simulink model "adc_nonlinconfig"  (R2013a)
settings: Solver=ode45  StartTime=0.0  StopTime=10e-05  RelTol=1e-3
undefined symbols (not defined in the file or in its folder): One, sided
libraries: dsparch4 x2, nonlinlib_config x1, dspsnks4 x1
settings Model: Creator=bbhattac  LastModifiedBy=bbhattac
settings OptimizationCC: ExpressionDepthLimit=2147483647
settings DebuggingCC: ParameterPrecisionLossMsg=none  FcnCallInpInsideContextMsg=UseLocalSettings
settings GRTTargetCC: CombineOutputUpdateFcns=off  GRTInterface=on

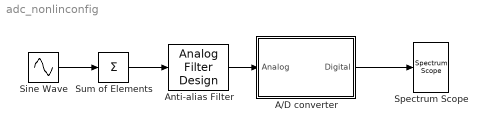
== system adc_nonlinconfig ==
  A/D converter : Subsystem
  Anti-alias Filter : dsparch4/Analog Filter Design  method=Butterworth  filttype=Lowpass  N=8  Wlo=2*pi*50e+06  Whi=80  Rp=2  Rs=40
  Sine Wave : Sin  Amplitude=.5  Frequency=2*pi*[20 22]*1e6  SampleTime=0
  Spectrum Scope : dspsnks4/Spectrum Scope  ScopeProperties=on  Domain=Frequency  HorizSpan=1  UseBuffer=on  BufferSize=2048  Overlap=0  TreatMby1Signals=M channels  inpFftLenInherit=off  FFTlength=128  numAvg=2  DisplayProperties=off  AxisGrid=on  Memory=off  FrameNumber=on  AxisLegend=off  AxisZoom=off  OpenScopeAtSimStart=on  OpenScopeImmediately=off  FigPos=[13 485 399 237]  AxisProperties=off  XUnits=Hertz  XRange=One-sided ([0...Fs/2])  XDisplay=0  InheritXIncr=on  XIncr=1.0  XLabel=Samples  XLimit=Auto  YUnits=dBW/Hertz  XMax=1  XMin=0  YLabel=Magnitude-squared, dB  LineProperties=off  wintypeSpecScope=Hann  RsSpecScope=50  betaSpecScope=5  winsampSpecScope=Periodic  XAxisParamsVer=6.9  isFrameUpgraded=on
      settings: YMin=-146.5665  YMax=-53.7967
  Sum of Elements : Sum  Inputs=+
  wires:
  Sine Wave/1 -> Sum of Elements/1
  Sum of Elements/1 -> Anti-alias Filter/1
  Anti-alias Filter/1 -> A/D converter/1(Analog)
  A/D converter/1(Digital) -> Spectrum Scope/1

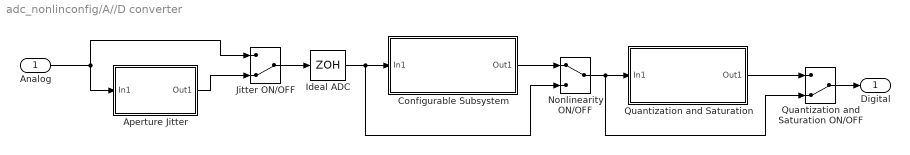
== system adc_nonlinconfig/A//D converter ==
  Analog : Inport
  Aperture Jitter : Subsystem
  Configurable Subsystem : Subsystem  BlockChoice=Lookup Table
      link override Nonlinearity-Sine: nonlingain=0.2
      link override Power Series Nonlinearity: nonlingain=1e-03
      settings: AttributesFormatString=%<BlockChoice>  TemplateBlock=nonlinlib_config/Configurable Subsystem  MemberBlocks=Dead Zone,Lookup Table,Nonlinearity-Sine,Nonlinearity-Tanh,Power Series Nonlinearity
  Ideal ADC : ZeroOrderHold  SampleTime=1/100e6
  Jitter ON/OFF : ManualSwitch  CurrentSetting=0
  Nonlinearity ON/OFF : ManualSwitch
  Quantization and Saturation ON/OFF : ManualSwitch  CurrentSetting=0
  Quantization and Saturation : Subsystem
  Digital : Outport
  wires:
  Analog/1 -> Jitter ON/OFF/1, Aperture Jitter/1(In1)
  Jitter ON/OFF/1 -> Ideal ADC/1
  Ideal ADC/1 -> Nonlinearity ON/OFF/2, Configurable Subsystem/1(In1)
  Quantization and Saturation/1(Out1) -> Quantization and Saturation ON/OFF/1
  Nonlinearity ON/OFF/1 -> Quantization and Saturation ON/OFF/2, Quantization and Saturation/1(In1)
  Configurable Subsystem/1(Out1) -> Nonlinearity ON/OFF/1
  Quantization and Saturation ON/OFF/1 -> Digital/1
  Aperture Jitter/1(Out1) -> Jitter ON/OFF/2

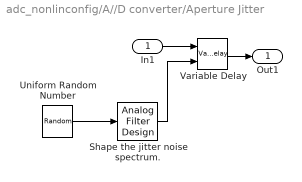
== system adc_nonlinconfig/A//D converter/Aperture Jitter ==
  In1 : Inport
  "Shape the jitter noise spectrum. " : dsparch4/Analog Filter Design  method=Butterworth  filttype=Lowpass  N=3  Wlo=2*pi*20e6  Whi=80  Rp=2  Rs=40
  Uniform Random Number : UniformRandomNumber  Minimum=0  Maximum=5e-9  Seed=1234  SampleTime=0
  Variable Delay : VariableTransportDelay  MaximumDelay=30e-9  ZeroDelay=on  TransDelayFeedthrough=on
  Out1 : Outport
  wires:
  Uniform Random Number/1 -> "Shape the jitter noise spectrum. "/1
  "Shape the jitter noise spectrum. "/1 -> Variable Delay/2
  In1/1 -> Variable Delay/1
  Variable Delay/1 -> Out1/1

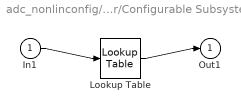
== system adc_nonlinconfig/A//D converter/Configurable Subsystem ==
  In1 : Inport
  Lookup Table : nonlinlib_config/Lookup Table  SystemSampleTime=-1
  Out1 : Outport
  wires:
  In1/1 -> Lookup Table/1
  Lookup Table/1 -> Out1/1

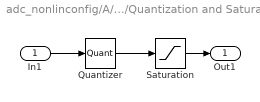
== system adc_nonlinconfig/A//D converter/Quantization and Saturation ==
  In1 : Inport
  Quantizer : Quantizer  QuantizationInterval=2^-8
  Saturation : Saturate  UpperLimit=1  LowerLimit=-1
  Out1 : Outport
  wires:
  Quantizer/1 -> Saturation/1
  In1/1 -> Quantizer/1
  Saturation/1 -> Out1/1
